simulink model "Assignment2"  (R2025b)
settings: Solver=ode45  StartTime=0.0  StopTime=5  MaxStep=1e-4  RelTol=1e-3
settings Model: Creator=57709  LastModifiedBy=57709

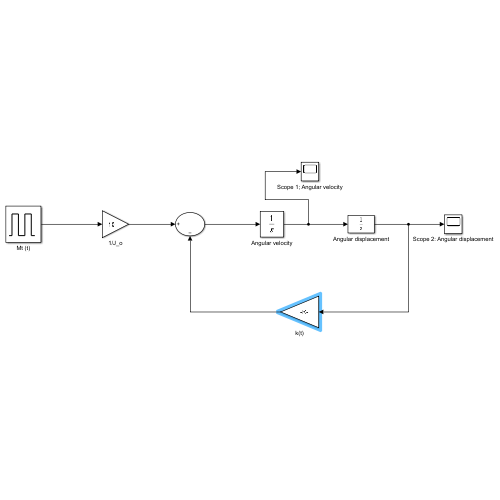
[thumbnail: Simulink's stored preview of the top-level diagram]
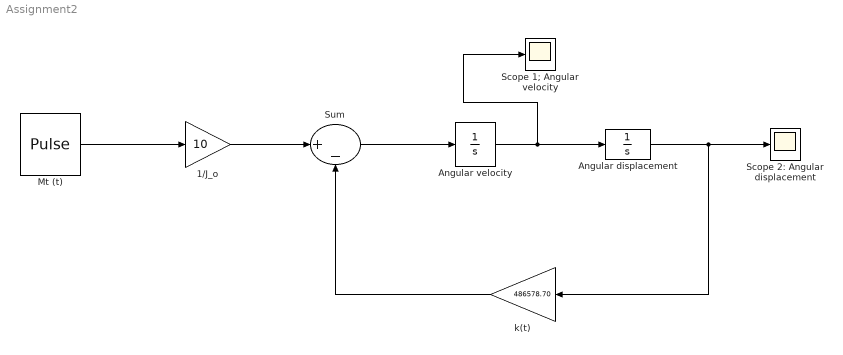
== system Assignment2 ==
  1/J_o : Gain  Gain=10
  Angular displacement : Integrator
  Angular velocity : Integrator
  Mt (t) : DiscretePulseGenerator  PulseType=Time based  Amplitude=1000  Period=0.06  PulseWidth=6.25
  Scope 1; Angular velocity : Scope
      settings: ActiveDisplayYMinimum=15.524039364324924  ActiveDisplayYMaximum=40.772729417491107
  Scope 2: Angular displacement : Scope
      settings: ActiveDisplayYMinimum=0.023203429988507371  ActiveDisplayYMaximum=0.054465577277599583
  Sum : Sum  Inputs=|+-
  k(t) : Gain  Gain=486578.70
  wires:
  Mt (t)/1 -> 1/J_o/1
  1/J_o/1 -> Sum/1
  Sum/1 -> Angular velocity/1
  Angular velocity/1 -> Scope 1; Angular velocity/1, Angular displacement/1
  Angular displacement/1 -> k(t)/1, Scope 2: Angular displacement/1
  k(t)/1 -> Sum/2
